simulink model "PID"  (R2023a)
settings: Solver=VariableStepAuto  StartTime=0.0  StopTime=10.0  RelTol=1e-3
settings Model: Creator=余嘉乐  LastModifiedBy=余嘉乐
settings DebuggingCC: AlgebraicLoopMsg=none

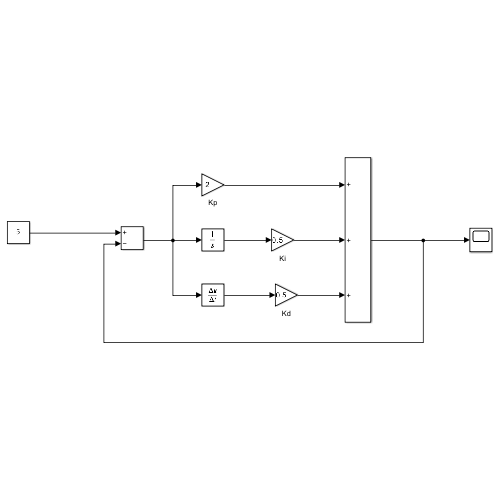
[thumbnail: Simulink's stored preview of the top-level diagram]
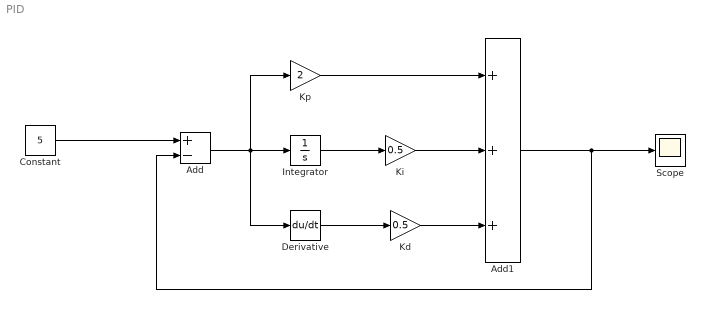
== system PID ==
  Add : Sum  Inputs=+-
  Add1 : Sum  Inputs=+++
  Constant : Constant  Value=5
  Derivative : Derivative
  Integrator : Integrator
  Kd : Gain  Gain=0.5
  Ki : Gain  Gain=0.5
  Kp : Gain  Gain=2
  Scope : Scope
  wires:
  Constant/1 -> Add/1
  Add/1 -> Derivative/1, Integrator/1, Kp/1
  Kp/1 -> Add1/1
  Integrator/1 -> Ki/1
  Derivative/1 -> Kd/1
  Add1/1 -> Add/2, Scope/1
  Ki/1 -> Add1/2
  Kd/1 -> Add1/3
